simulink model "ad9361_sim"  (R2014b)
settings: Solver=ode45  StartTime=0.0  StopTime=Inf  RelTol=1e-3
libraries: simulink x1
settings Model: Creator=ACozma  LastModifiedBy=DPu1
settings DataIOCC: SignalLoggingSaveFormat=ModelDataLogs
settings DebuggingCC: UnderspecifiedInitializationDetection=Classic  MergeDetectMultiDrivingBlocksExec=none  MultiTaskDSMMsg=warning  MultiTaskCondExecSysMsg=none
settings RTWCC: IncludeERTFirstTime=on

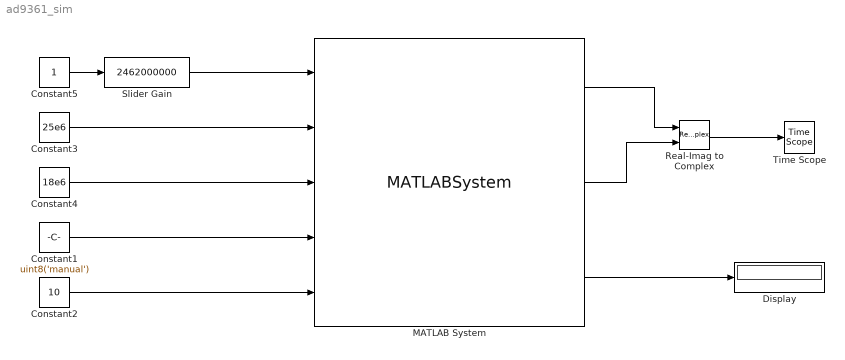
== system ad9361_sim ==
  Constant1 : Constant  Value=uint8('manual')  SampleTime=1
  Constant2 : Constant  Value=10  SampleTime=1
  Constant3 : Constant  Value=25e6  SampleTime=1
  Constant4 : Constant  Value=18e6  SampleTime=1
  Constant5 : Constant  SampleTime=1
  Display : Display
  MATLAB System : MATLABSystem  System=iio_sys_obj  SimulateUsing=Interpreted execution  ip_address=10.66.99.53  dev_name=ad9361  in_ch_no=0  in_ch_size=32768  out_ch_no=2  out_ch_size=8192
      mask Type: iio_sys_obj
      mask Display:
      | disp('ad9361');
      | port_label('input',1,'RX_LO_FREQ');
      | port_label('input',2,'RX_SAMPLING_FREQ');
      | port_label('input',3,'RX_RF_BANDWIDTH');
      | port_label('input',4,'RX1_GAIN_MODE');
      | port_label('input',5,'RX1_GAIN');
      | port_label('output',1,'DATA_OUT1');
      | port_label('output',2,'DATA_OUT2');
      | port_label('output',3,'RX1_RSSI');
  Real-Imag to Complex : RealImagToComplex
  Slider Gain : simulink/Math Operations/Slider Gain  low=200000  gain=2462000000  high=6000000000
  Time Scope : TimeScope  DefaultConfigurationName=spbscopes.TimeScopeBlockCfg
  wires:
  Constant5/1 -> Slider Gain/1
  MATLAB System/1 -> Real-Imag to Complex/1
  Real-Imag to Complex/1 -> Time Scope/1
  Slider Gain/1 -> MATLAB System/1
  Constant3/1 -> MATLAB System/2
  Constant4/1 -> MATLAB System/3
  Constant1/1 -> MATLAB System/4
  Constant2/1 -> MATLAB System/5
  MATLAB System/3 -> Display/1
  MATLAB System/2 -> Real-Imag to Complex/2
